simulink model "sim_final_VSS_PWM"  (R2019a)
settings: Solver=ode8  StartTime=0.0  StopTime=end_time  FixedStep=FStep  RelTol=1e-3  EnableMultiTasking=on
values from neighbouring files (symbols this model uses):
  a = av(i)    [R2018b.m]
  Am = d    [R2018b.m]
  b = bv(i)    [R2018b.m]
  C1 = C1v(i)    [R2018b.m]
  C2 = C2v(i)    [R2018b.m]
  d = InitialConditions.d    [R2018b.m]
  ds = 1    [R2018b.m]
  h = InitialConditions.h    [R2018b.m]
  K = InitialConditions.K    [R2018b.m]
  k1 = k1v(i)    [R2018b.m]
  k2 = k2v(i)    [R2018b.m]
  sw1 = sw1v(2)    [R2018b.m]
  T = InitialConditions.T    [R2018b.m]
  Ts = Tsv(i)    [R2018b.m]
  x0 = 0    [R2018b.m]
  y0 = 0    [R2018b.m]
  z0 = 0    [R2018b.m]
  zad = 100    [R2018b.m]
libraries: simulink x2, simulink_extras x1
settings Model: Creator=user  LastModifiedBy=ogure
settings SolverCC: SolverResetMethod=Robust  AutoInsertRateTranBlk=on
settings DataIOCC: LimitDataPoints=on  SaveFormat=Array  SaveOutput=off  ReturnWorkspaceOutputs=off  OutputSaveName=X,X1,X2,X3,X4,L,H
settings OptimizationCC: LifeSpan=inf
settings DebuggingCC: SolverPrmCheckMsg=warning  SFUnexpectedBacktrackingDiag=warning  SFNoUnconditionalDefaultTransitionDiag=warning  SFExecutionAtInitializationDiag=none  ArithmeticOperatorsInVariantConditions=warning
settings HardwareCC: ProdBitPerPointer=32  ProdBitPerSizeT=32  ProdBitPerPtrDiffT=32  ProdLargestAtomicFloat=None  ProdIntDivRoundTo=Undefined  ProdEndianess=Unspecified  ProdWordSize=32  ProdHWDeviceType=32-bit Generic
settings ModelReferenceCC: PropagateSignalLabelsOutOfModel=off
settings SFSimCC: SimUseLocalCustomCode=off
settings RTWCC: RTWUseLocalCustomCode=off
settings CodeAppCC: StateflowObjectComments=on
settings GRTTargetCC: TargetLangStandard=C89/C90 (ANSI)  GeneratePreprocessorConditionals=Disable all
settings ConfigComp: CovMetricSettings=dw  CovHtmlReporting=on  CovSaveCumulativeToWorkspaceVar=on  CovSaveSingleToWorkspaceVar=on  CovExternalEMLEnable=off  CovSFcnEnable=off

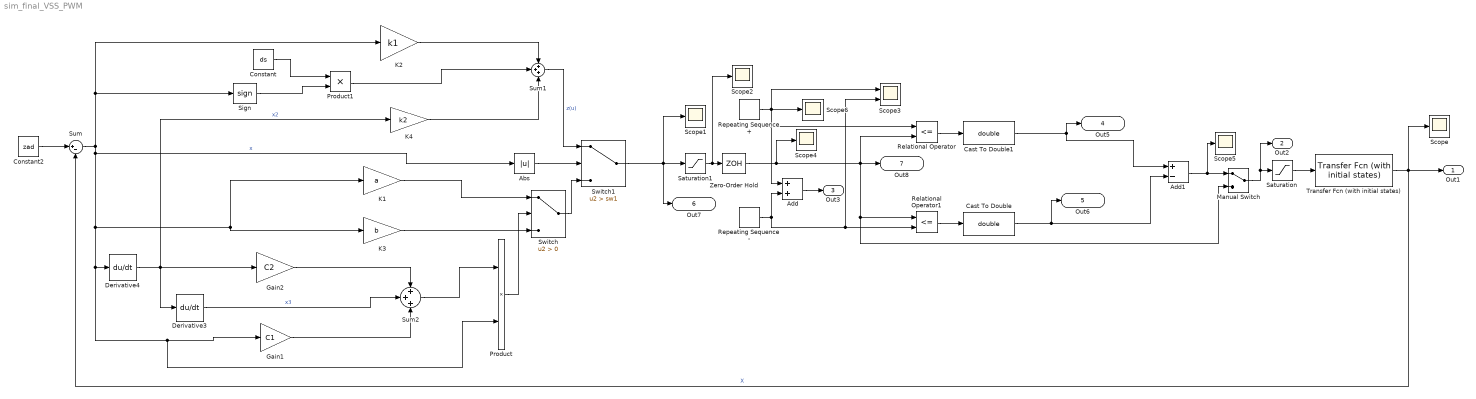
== system sim_final_VSS_PWM ==
  Abs : Abs
  Add : Sum
  Add1 : Sum  Inputs=+-
  Cast To Double : DataTypeConversion  OutDataTypeStr=double
  Cast To Double1 : DataTypeConversion  OutDataTypeStr=double
  Constant : Constant  Value=ds
  Constant2 : Constant  Value=zad
  Derivative3 : Derivative  CoefficientInTFapproximation=0.00000001
  Derivative4 : Derivative  CoefficientInTFapproximation=0.00000001
  Gain1 : Gain  Gain=C1
  Gain2 : Gain  Gain=C2
  K1 : Gain  Gain=a
  K2 : Gain  Gain=k1
  K3 : Gain  Gain=b
  K4 : Gain  Gain=k2
  Manual Switch : ManualSwitch
  Product : Product
  Product1 : Product
  Relational Operator : RelationalOperator  Operator=<=  OutDataTypeStr=boolean  ZeroCross=off  RndMeth=Simplest
  Relational Operator1 : RelationalOperator  Operator=<=  OutDataTypeStr=boolean  ZeroCross=off  RndMeth=Simplest
  Repeating Sequence + : simulink/Sources/Repeating Sequence  rep_seq_t=[0 Ts]  rep_seq_y=[0 Am]
  Repeating Sequence - : simulink/Sources/Repeating Sequence  rep_seq_t=[0 Ts]  rep_seq_y=[0 -Am]
  Saturation : Saturate  UpperLimit=d  LowerLimit=-d
  Saturation1 : Saturate  UpperLimit=d  LowerLimit=-d
  Scope{,1..2,4..6} (6 alike) : Scope
  Scope3 : Scope  NumInputPorts=2
  Sign : Signum
  Sum : Sum  Inputs=|+-
  Sum1 : Sum  Inputs=+++
  Sum2 : Sum  Inputs=+++
  Switch : Switch  Criteria=u2 > Threshold  ZeroCross=off
  Switch1 : Switch  Criteria=u2 > Threshold  Threshold=sw1  ZeroCross=off
  Transfer Fcn (with initial states) : simulink_extras/Additional Linear/Transfer Fcn (with initial states)  N=K  D=[T^2 2*h*T 1 0]  X0=[z0 y0 x0]
  Zero-Order Hold : ZeroOrderHold  SampleTime=Ts
  Out1 : Outport  SignalName=X
  Out2 : Outport  Port=2  SignalName=PWm
  Out3 : Outport  Port=3  SignalName=saw
  Out5 : Outport  Port=4  SignalName=pwm1
  Out6 : Outport  Port=5  SignalName=pwm2
  Out7 : Outport  Port=6  SignalName=upr
  Out8 : Outport  Port=7  SignalName=upr_ogr
  wires:
  Transfer Fcn (with initial states)/1 -> Scope/1, Sum/2, Out1/1  "X"
  Derivative3/1 -> Sum2/2  "x3"
  Gain1/1 -> Sum2/3
  Sum2/1 -> Product/1
  K1/1 -> Switch/1
  Sum/1 -> Abs/1, K1/1, K3/1, Gain1/1, Product/2, Derivative4/1, K2/1, Sign/1  "x"
  Derivative4/1 -> K4/1, Gain2/1, Derivative3/1  "x2"
  Product/1 -> Switch/2
  Gain2/1 -> Sum2/1
  K3/1 -> Switch/3
  Switch/1 -> Switch1/3
  Sign/1 -> Product1/2
  Constant/1 -> Product1/1
  K2/1 -> Sum1/1
  K4/1 -> Sum1/3
  Product1/1 -> Sum1/2
  Constant2/1 -> Sum/1
  Sum1/1 -> Switch1/1  "z(u)"
  Abs/1 -> Switch1/2
  Cast To Double1/1 -> Add1/1, Out5/1
  Cast To Double/1 -> Add1/2, Out6/1
  Saturation1/1 -> Scope2/1, Zero-Order Hold/1
  Zero-Order Hold/1 -> Scope4/1, Relational Operator1/1, Manual Switch/2, Out8/1, Relational Operator/2
  Repeating Sequence -/1 -> Add/2, Scope3/2, Relational Operator1/2
  Repeating Sequence +/1 -> Add/1, Relational Operator/1, Scope3/1, Scope6/1
  Saturation/1 -> Transfer Fcn (with initial states)/1
  Switch1/1 -> Scope1/1, Out7/1, Saturation1/1
  Add1/1 -> Scope5/1, Manual Switch/1
  Relational Operator/1 -> Cast To Double1/1
  Relational Operator1/1 -> Cast To Double/1
  Add/1 -> Out3/1
  Manual Switch/1 -> Out2/1, Saturation/1
